simulink model "FFT"  (R2021a)
settings: Solver=VariableStepAuto  StartTime=0.0  StopTime=10.0  RelTol=1e-3
libraries: dspxfrm3 x1
settings Model: Creator=LEGION  LastModifiedBy=LEGION

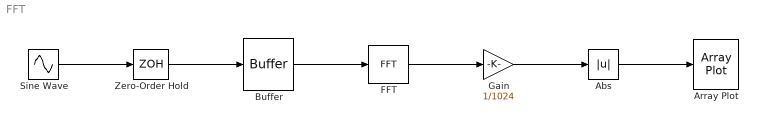
== system FFT ==
  Abs : Abs
  Array Plot : ArrayPlot  WindowPosition=[94.000000,350.000000,800.000000,500.000000,]  MaximizeAxes=Off  YLimits=[0.0034744617327237257,0.004852178417895007]  DefaultConfigurationName=dsp.scopes.ArrayPlotBlockSpecification
  Buffer : Buffer  N=1024  OutputFrames=off
  FFT : dspxfrm3/FFT  FFTImplementation=Auto  CompMethod=Table lookup  TableOpt=NEW  TableOptActive=Speed  BitRevOrder=off  Normalize=off  InheritFFTLength=on  FFTLength=64  WrapInput=on  roundingMode=Floor  overflowMode=off  firstCoeffDataTypeStr=Inherit: Same word length as input  firstCoeffLastDataTypeStr=Inherit: Same word length as input  outputMin=[]  outputMax=[]
  Gain : Gain  Gain=1/1024
  Sine Wave : Sin  Amplitude=8  Frequency=2*pi*1e3  SampleTime=0
  Zero-Order Hold : ZeroOrderHold  SampleTime=1e-5
  wires:
  Sine Wave/1 -> Zero-Order Hold/1
  Zero-Order Hold/1 -> Buffer/1
  Buffer/1 -> FFT/1
  FFT/1 -> Gain/1
  Gain/1 -> Abs/1
  Abs/1 -> Array Plot/1
